simulink model "P1_GeneralizedPlant_RS_NP"  (R2024b)
settings: Solver=VariableStepAuto  StartTime=0.0  StopTime=10.0  RelTol=1e-3
values from neighbouring files (symbols this model uses):
  Ga = 0.095    [P1.m]
libraries: cstblocks x3
settings Model: Creator=lucap  LastModifiedBy=lucap

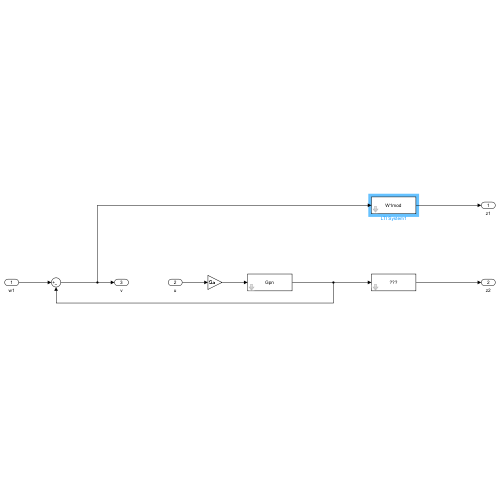
[thumbnail: Simulink's stored preview of the top-level diagram]
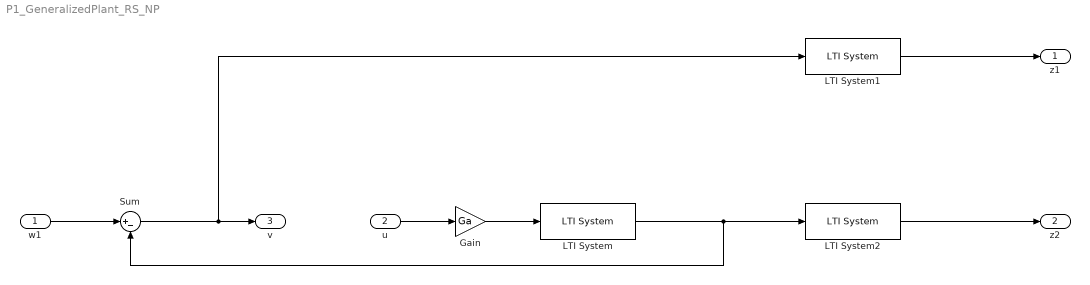
== system P1_GeneralizedPlant_RS_NP ==
  w1 : Inport
  u : Inport  Port=2
  Gain : Gain  Gain=Ga
  LTI System : cstblocks/LTI System  sys=Gpn  IC=[]  PadeOrder=0
  LTI System1 : cstblocks/LTI System  sys=W1mod  IC=[]  PadeOrder=0
  LTI System2 : cstblocks/LTI System  sys=W2mod  IC=[]  PadeOrder=0
  Sum : Sum  Inputs=|+-
  z1 : Outport
  z2 : Outport  Port=2
  v : Outport  Port=3
  wires:
  w1/1 -> Sum/1
  LTI System1/1 -> z1/1
  LTI System2/1 -> z2/1
  Gain/1 -> LTI System/1
  u/1 -> Gain/1
  Sum/1 -> v/1, LTI System1/1
  LTI System/1 -> LTI System2/1, Sum/2
